simulink library "INT_RailP_DD"  (R2016b)
settings: Solver=VariableStepAuto  StartTime=0.0  StopTime=10.0  RelTol=1e-3
settings Model: Creator=liangyunbo  LastModifiedBy=liangyunbo

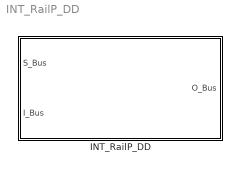
== system INT_RailP_DD ==
  INT_RailP_DD : Subsystem

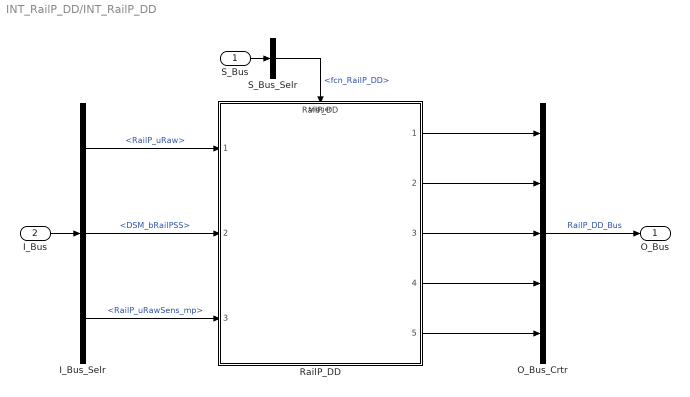
== system INT_RailP_DD/INT_RailP_DD ==
  S_Bus : Inport
  I_Bus : Inport  Port=2
  I_Bus_Selr : BusSelector  OutputSignals=RailP_uRaw,DSM_bRailPSS,RailP_uRawSens_mp
  O_Bus_Crtr : BusCreator  Inputs=5
  RailP_DD : ModelReference  ModelNameDialog=RailP_DD  SimulationMode=Normal  ModelReferenceVersion=1.29  TriggerPortName=function  TriggerPortTriggerType=function-call  TriggerPortStatesWhenEnabling=held
  S_Bus_Selr : BusSelector  OutputSignals=fcn_RailP_DD
  O_Bus : Outport
  wires:
  S_Bus_Selr/1 -> RailP_DD/Trigger  "<fcn_RailP_DD>"
  S_Bus/1 -> S_Bus_Selr/1
  I_Bus/1 -> I_Bus_Selr/1
  I_Bus_Selr/1 -> RailP_DD/1  "<RailP_uRaw>"
  I_Bus_Selr/2 -> RailP_DD/2  "<DSM_bRailPSS>"
  I_Bus_Selr/3 -> RailP_DD/3  "<RailP_uRawSens_mp>"
  O_Bus_Crtr/1 -> O_Bus/1  "RailP_DD_Bus"
  RailP_DD/1 -> O_Bus_Crtr/1
  RailP_DD/2 -> O_Bus_Crtr/2
  RailP_DD/3 -> O_Bus_Crtr/3
  RailP_DD/4 -> O_Bus_Crtr/4
  RailP_DD/5 -> O_Bus_Crtr/5
